simulink library "sm_wheel_loader_lib"  (R2026a)
settings: Solver=VariableStepAuto
undefined symbols (not defined in the file): AToTOrificeVector, BiPOrificeVector, boomHEArea, boomREArea, BToTOrificeVector, fluids, GRake, GToothL, GToothR, HMPST, HydFcnParams, logLoad, Position, PToAOrificeVector, PToBOrificeVector, RakeL, RakeR, testInput, Wheel_Loader, X, Y, Z
libraries: sm_lib x694, fl_lib x183, nesl_utility x74, SimscapeFluids_lib x62, sdl_lib x25, cvt_components_lib x25, simulink_extras x5, $bdroot x4, wheel_loader_contact_lib x4, ee_lib x2, SignalEditorBlockLib x1, batteryecm_lib x1
(part 9 of 25)

== system sm_wheel_loader_lib/Wheel Loader Vehicle/Steering Actuator/Cylinder ==
  Collar : sm_lib/Body Elements/File Solid  ExtGeomFileName=Steer_Act_Cylinder_Collar.STEP  UnitType=FromFile  ExtGeomFileUnits=m  StepReaderType=HEX  ExportConvexHullGeometry=off  InertiaType=Custom  BasedOnType=DensityFromFile  Density=1000  DensityUnits=kg/m^3  Mass=Wheel_Loader.bodyGroups(50).subGroups(3).inertialProperties.mass  MassUnits=kg  CenterOfMass=Wheel_Loader.bodyGroups(50).subGroups(3).inertialProperties.centerOfMass  CenterOfMassUnits=m  MomentsOfInertia=Wheel_Loader.bodyGroups(50).subGroups(3).inertialProperties.momentsOfInertia  MomentsOfInertiaUnits=kg*m^2  ProductsOfInertia=Wheel_Loader.bodyGroups(50).subGroups(3).inertialProperties.productsOfInertia  ProductsOfInertiaUnits=kg*m^2  GraphicType=FromGeometry  MarkerShape=Sphere  MarkerSize=10  GraphicVisPropType=SimpleVisualProperties  GraphicDiffuseColor=Wheel_Loader.bodyGroups(50).subGroups(3).visualProperties.rgb  GraphicOpacity=Wheel_Loader.bodyGroups(50).subGroups(3).visualProperties.opacity  GraphicSpecularColor=[0.5 0.5 0.5 1.0]  GraphicAmbientColor=[0.15 0.15 0.15 1.0]  GraphicEmissiveColor=[0.0 0.0 0.0 1.0]  GraphicShininess=75  DoExposeReferenceFrame=on  SerializedFrames=<Frames/>
  Cylinder : sm_lib/Body Elements/File Solid  ExtGeomFileName=Steer_Act_Cylinder.STEP  UnitType=FromFile  ExtGeomFileUnits=m  StepReaderType=HEX  ExportConvexHullGeometry=off  InertiaType=Custom  BasedOnType=DensityFromFile  Density=1000  DensityUnits=kg/m^3  Mass=Wheel_Loader.bodyGroups(50).subGroups(1).inertialProperties.mass  MassUnits=kg  CenterOfMass=Wheel_Loader.bodyGroups(50).subGroups(1).inertialProperties.centerOfMass  CenterOfMassUnits=m  MomentsOfInertia=Wheel_Loader.bodyGroups(50).subGroups(1).inertialProperties.momentsOfInertia  MomentsOfInertiaUnits=kg*m^2  ProductsOfInertia=Wheel_Loader.bodyGroups(50).subGroups(1).inertialProperties.productsOfInertia  ProductsOfInertiaUnits=kg*m^2  GraphicType=FromGeometry  MarkerShape=Sphere  MarkerSize=10  GraphicVisPropType=SimpleVisualProperties  GraphicDiffuseColor=Wheel_Loader.bodyGroups(50).subGroups(1).visualProperties.rgb  GraphicOpacity=Wheel_Loader.bodyGroups(50).subGroups(1).visualProperties.opacity  GraphicSpecularColor=[0.5 0.5 0.5 1.0]  GraphicAmbientColor=[0.15 0.15 0.15 1.0]  GraphicEmissiveColor=[0.0 0.0 0.0 1.0]  GraphicShininess=75  DoExposeReferenceFrame=on  SerializedFrames=<Frames/>
  RT_RearFrame_SteeringActCyl : sm_lib/Frames and Transforms/Rigid Transform  RotationMethod=RotationMatrix  FollAlignAxisA=+X  BaseAlignAxisA=+Y  FollAlignAxisB=+Y  BaseAlignAxisB=+Z  RotationStandardAxis=+Z  RotationAngle=0.0  RotationAngleUnits=deg  RotationArbitraryAxis=[0 0 1]  RotationSequenceAxes=FollowerAxes  RotationSequence=XYX  RotationSequenceAngles=[0 0 0]  RotationSequenceAnglesUnits=deg  RotationMatrix=Wheel_Loader.coordSys(23).transform.rotation  Quaternion=[1 0 0 0]  TranslationMethod=Cartesian  TranslationCartesianOffset=Wheel_Loader.coordSys(23).transform.translation  TranslationCartesianOffsetUnits=m  TranslationStandardAxis=+Z  TranslationStandardOffset=0  TranslationStandardOffsetUnits=m  TranslationROffset=0  TranslationROffsetUnits=m  TranslationThetaOffset=0  TranslationThetaOffsetUnits=deg  TranslationZOffset=0  TranslationZOffsetUnits=m
  RT_Steering_Actuator : sm_lib/Frames and Transforms/Rigid Transform  RotationMethod=RotationMatrix  FollAlignAxisA=+X  BaseAlignAxisA=+Y  FollAlignAxisB=+Y  BaseAlignAxisB=+Z  RotationStandardAxis=+Z  RotationAngle=0.0  RotationAngleUnits=deg  RotationArbitraryAxis=[0 0 1]  RotationSequenceAxes=FollowerAxes  RotationSequence=XYX  RotationSequenceAngles=[0 0 0]  RotationSequenceAnglesUnits=deg  RotationMatrix=Wheel_Loader.coordSys(24).transform.rotation  Quaternion=[1 0 0 0]  TranslationMethod=Cartesian  TranslationCartesianOffset=Wheel_Loader.coordSys(24).transform.translation  TranslationCartesianOffsetUnits=m  TranslationStandardAxis=+Z  TranslationStandardOffset=0  TranslationStandardOffsetUnits=m  TranslationROffset=0  TranslationROffsetUnits=m  TranslationThetaOffset=0  TranslationThetaOffsetUnits=deg  TranslationZOffset=0  TranslationZOffsetUnits=m
  RT_Steering_Actuator_Offset : sm_lib/Frames and Transforms/Rigid Transform  RotationMethod=None  FollAlignAxisA=+X  BaseAlignAxisA=+Y  FollAlignAxisB=+Y  BaseAlignAxisB=+Z  RotationStandardAxis=+Z  RotationAngle=0.0  RotationAngleUnits=deg  RotationArbitraryAxis=[0 0 1]  RotationSequenceAxes=FollowerAxes  RotationSequence=XYX  RotationSequenceAngles=[0 0 0]  RotationSequenceAnglesUnits=deg  RotationMatrix=[1 0 0; 0 1 0; 0 0 1]  Quaternion=[1 0 0 0]  TranslationMethod=StandardAxis  TranslationCartesianOffset=[0 0 0]  TranslationCartesianOffsetUnits=m  TranslationStandardAxis=+Z  TranslationStandardOffset=HydFcnParams.steerActuator.mechModelCylOffset  TranslationStandardOffsetUnits=mm  TranslationROffset=0  TranslationROffsetUnits=m  TranslationThetaOffset=0  TranslationThetaOffsetUnits=deg  TranslationZOffset=0  TranslationZOffsetUnits=m
  Seal : sm_lib/Body Elements/File Solid  ExtGeomFileName=Steer_Act_Cylinder_Seal.STEP  UnitType=FromFile  ExtGeomFileUnits=m  StepReaderType=HEX  ExportConvexHullGeometry=off  InertiaType=Custom  BasedOnType=DensityFromFile  Density=1000  DensityUnits=kg/m^3  Mass=Wheel_Loader.bodyGroups(50).subGroups(2).inertialProperties.mass  MassUnits=kg  CenterOfMass=Wheel_Loader.bodyGroups(50).subGroups(2).inertialProperties.centerOfMass  CenterOfMassUnits=m  MomentsOfInertia=Wheel_Loader.bodyGroups(50).subGroups(2).inertialProperties.momentsOfInertia  MomentsOfInertiaUnits=kg*m^2  ProductsOfInertia=Wheel_Loader.bodyGroups(50).subGroups(2).inertialProperties.productsOfInertia  ProductsOfInertiaUnits=kg*m^2  GraphicType=FromGeometry  MarkerShape=Sphere  MarkerSize=10  GraphicVisPropType=SimpleVisualProperties  GraphicDiffuseColor=Wheel_Loader.bodyGroups(50).subGroups(2).visualProperties.rgb  GraphicOpacity=Wheel_Loader.bodyGroups(50).subGroups(2).visualProperties.opacity  GraphicSpecularColor=[0.5 0.5 0.5 1.0]  GraphicAmbientColor=[0.15 0.15 0.15 1.0]  GraphicEmissiveColor=[0.0 0.0 0.0 1.0]  GraphicShininess=75  DoExposeReferenceFrame=on  SerializedFrames=<Frames/>
  B : PMIOPort  Side=Left
  F : PMIOPort  Port=2  Side=Right
  connections:
  Seal/RConn1 -- Collar/RConn1 -- Cylinder/RConn1 -- RT_RearFrame_SteeringActCyl/LConn1 -- RT_Steering_Actuator/LConn1
  RT_RearFrame_SteeringActCyl/RConn1 -- B/RConn1
  RT_Steering_Actuator_Offset/RConn1 -- F/RConn1
  RT_Steering_Actuator/RConn1 -- RT_Steering_Actuator_Offset/LConn1

== system sm_wheel_loader_lib/Wheel Loader Vehicle/Steering Actuator/Rod ==
  Collar : sm_lib/Body Elements/File Solid  ExtGeomFileName=Steer_Act_Rod_Collar.STEP  UnitType=FromFile  ExtGeomFileUnits=m  StepReaderType=HEX  ExportConvexHullGeometry=off  InertiaType=Custom  BasedOnType=DensityFromFile  Density=1000  DensityUnits=kg/m^3  Mass=Wheel_Loader.bodyGroups(51).subGroups(2).inertialProperties.mass  MassUnits=kg  CenterOfMass=Wheel_Loader.bodyGroups(51).subGroups(2).inertialProperties.centerOfMass  CenterOfMassUnits=m  MomentsOfInertia=Wheel_Loader.bodyGroups(51).subGroups(2).inertialProperties.momentsOfInertia  MomentsOfInertiaUnits=kg*m^2  ProductsOfInertia=Wheel_Loader.bodyGroups(51).subGroups(2).inertialProperties.productsOfInertia  ProductsOfInertiaUnits=kg*m^2  GraphicType=FromGeometry  MarkerShape=Sphere  MarkerSize=10  GraphicVisPropType=SimpleVisualProperties  GraphicDiffuseColor=Wheel_Loader.bodyGroups(51).subGroups(2).visualProperties.rgb  GraphicOpacity=Wheel_Loader.bodyGroups(51).subGroups(2).visualProperties.opacity  GraphicSpecularColor=[0.5 0.5 0.5 1.0]  GraphicAmbientColor=[0.15 0.15 0.15 1.0]  GraphicEmissiveColor=[0.0 0.0 0.0 1.0]  GraphicShininess=75  DoExposeReferenceFrame=on  SerializedFrames=<Frames/>
  RT_SteeringActRod_FrontFrame : sm_lib/Frames and Transforms/Rigid Transform  RotationMethod=RotationMatrix  FollAlignAxisA=+X  BaseAlignAxisA=+Y  FollAlignAxisB=+Y  BaseAlignAxisB=+Z  RotationStandardAxis=+Z  RotationAngle=0.0  RotationAngleUnits=deg  RotationArbitraryAxis=[0 0 1]  RotationSequenceAxes=FollowerAxes  RotationSequence=XYX  RotationSequenceAngles=[0 0 0]  RotationSequenceAnglesUnits=deg  RotationMatrix=Wheel_Loader.coordSys(25).transform.rotation  Quaternion=[1 0 0 0]  TranslationMethod=Cartesian  TranslationCartesianOffset=Wheel_Loader.coordSys(25).transform.translation  TranslationCartesianOffsetUnits=m  TranslationStandardAxis=+Z  TranslationStandardOffset=0  TranslationStandardOffsetUnits=m  TranslationROffset=0  TranslationROffsetUnits=m  TranslationThetaOffset=0  TranslationThetaOffsetUnits=deg  TranslationZOffset=0  TranslationZOffsetUnits=m
  RT_Steering_Actuator : sm_lib/Frames and Transforms/Rigid Transform  RotationMethod=RotationMatrix  FollAlignAxisA=+X  BaseAlignAxisA=+Y  FollAlignAxisB=+Y  BaseAlignAxisB=+Z  RotationStandardAxis=+Z  RotationAngle=0.0  RotationAngleUnits=deg  RotationArbitraryAxis=[0 0 1]  RotationSequenceAxes=FollowerAxes  RotationSequence=XYX  RotationSequenceAngles=[0 0 0]  RotationSequenceAnglesUnits=deg  RotationMatrix=Wheel_Loader.coordSys(24).transform.rotation  Quaternion=[1 0 0 0]  TranslationMethod=Cartesian  TranslationCartesianOffset=Wheel_Loader.coordSys(24).transform.translation  TranslationCartesianOffsetUnits=m  TranslationStandardAxis=+Z  TranslationStandardOffset=0  TranslationStandardOffsetUnits=m  TranslationROffset=0  TranslationROffsetUnits=m  TranslationThetaOffset=0  TranslationThetaOffsetUnits=deg  TranslationZOffset=0  TranslationZOffsetUnits=m
  RT_Steering_Actuator_Offset : sm_lib/Frames and Transforms/Rigid Transform  RotationMethod=None  FollAlignAxisA=+X  BaseAlignAxisA=+Y  FollAlignAxisB=+Y  BaseAlignAxisB=+Z  RotationStandardAxis=+Z  RotationAngle=0.0  RotationAngleUnits=deg  RotationArbitraryAxis=[0 0 1]  RotationSequenceAxes=FollowerAxes  RotationSequence=XYX  RotationSequenceAngles=[0 0 0]  RotationSequenceAnglesUnits=deg  RotationMatrix=[1 0 0; 0 1 0; 0 0 1]  Quaternion=[1 0 0 0]  TranslationMethod=StandardAxis  TranslationCartesianOffset=[0 0 0]  TranslationCartesianOffsetUnits=m  TranslationStandardAxis=+Z  TranslationStandardOffset=HydFcnParams.steerActuator.mechModelRodOffset  TranslationStandardOffsetUnits=mm  TranslationROffset=0  TranslationROffsetUnits=m  TranslationThetaOffset=0  TranslationThetaOffsetUnits=deg  TranslationZOffset=0  TranslationZOffsetUnits=m
  Rod : sm_lib/Body Elements/File Solid  ExtGeomFileName=Steer_Act_Rod.STEP  UnitType=FromFile  ExtGeomFileUnits=m  StepReaderType=HEX  ExportConvexHullGeometry=off  InertiaType=Custom  BasedOnType=DensityFromFile  Density=1000  DensityUnits=kg/m^3  Mass=Wheel_Loader.bodyGroups(51).subGroups(1).inertialProperties.mass  MassUnits=kg  CenterOfMass=Wheel_Loader.bodyGroups(51).subGroups(1).inertialProperties.centerOfMass  CenterOfMassUnits=m  MomentsOfInertia=Wheel_Loader.bodyGroups(51).subGroups(1).inertialProperties.momentsOfInertia  MomentsOfInertiaUnits=kg*m^2  ProductsOfInertia=Wheel_Loader.bodyGroups(51).subGroups(1).inertialProperties.productsOfInertia  ProductsOfInertiaUnits=kg*m^2  GraphicType=FromGeometry  MarkerShape=Sphere  MarkerSize=10  GraphicVisPropType=SimpleVisualProperties  GraphicDiffuseColor=Wheel_Loader.bodyGroups(51).subGroups(1).visualProperties.rgb  GraphicOpacity=Wheel_Loader.bodyGroups(51).subGroups(1).visualProperties.opacity  GraphicSpecularColor=[0.5 0.5 0.5 1.0]  GraphicAmbientColor=[0.15 0.15 0.15 1.0]  GraphicEmissiveColor=[0.0 0.0 0.0 1.0]  GraphicShininess=75  DoExposeReferenceFrame=on  SerializedFrames=<Frames/>
  B : PMIOPort  Side=Left
  F : PMIOPort  Port=2  Side=Right
  connections:
  RT_Steering_Actuator/LConn1 -- Collar/RConn1 -- Rod/RConn1 -- RT_SteeringActRod_FrontFrame/LConn1
  RT_Steering_Actuator_Offset/RConn1 -- B/RConn1
  RT_SteeringActRod_FrontFrame/RConn1 -- F/RConn1
  RT_Steering_Actuator/RConn1 -- RT_Steering_Actuator_Offset/LConn1

== system sm_wheel_loader_lib/Controller/Desired Ratio Calc/HRB Control/PI HRB Brake ==
  error : Inport
  Rset : Inport  Port=2
  Gain : Gain  Gain=0.02*0.2
  Gain3 : Gain  Gain=0.002+0.0005
  Integrator : Integrator  ExternalReset=falling
  Sum : Sum  Inputs=++|
  ctrl : Outport
  wires:
  Rset/1 -> Integrator/2
  Integrator/1 -> Sum/1
  error/1 -> Gain3/1, Gain/1
  Sum/1 -> ctrl/1
  Gain3/1 -> Integrator/1
  Gain/1 -> Sum/2

== system sm_wheel_loader_lib/Controller/Desired Ratio Calc/HRB Control/PI HRB Regen ==
  error : Inport
  Rset : Inport  Port=2
  Gain : Gain  Gain=0.01*0.2
  Gain3 : Gain  Gain=0.001
  Integrator : Integrator  ExternalReset=falling
  Sum : Sum  Inputs=++|
  ctrl : Outport
  wires:
  Gain/1 -> Sum/2
  Gain3/1 -> Integrator/1
  Sum/1 -> ctrl/1
  error/1 -> Gain/1, Gain3/1
  Integrator/1 -> Sum/1
  Rset/1 -> Integrator/2

== system sm_wheel_loader_lib/Controller/Desired Ratio Calc/MB Control/PI MB No HRB ==
  error : Inport
  Rset : Inport  Port=2
  Gain : Gain  Gain=0.01
  Gain3 : Gain  Gain=0.002
  Integrator : Integrator  ExternalReset=falling
  Sum : Sum  Inputs=++|
  ctrl : Outport
  wires:
  Rset/1 -> Integrator/2
  Integrator/1 -> Sum/1
  error/1 -> Gain3/1, Gain/1
  Sum/1 -> ctrl/1
  Gain3/1 -> Integrator/1
  Gain/1 -> Sum/2

== system sm_wheel_loader_lib/Controller/Desired Ratio Calc/MB Control/PI MB with MRB ==
  error : Inport
  Rset : Inport  Port=2
  Gain : Gain  Gain=0.005
  Gain3 : Gain  Gain=0.002
  Integrator : Integrator  ExternalReset=falling
  Sum : Sum  Inputs=++|
  ctrl : Outport
  wires:
  Gain/1 -> Sum/2
  Gain3/1 -> Integrator/1
  Sum/1 -> ctrl/1
  error/1 -> Gain/1, Gain3/1
  Integrator/1 -> Sum/1
  Rset/1 -> Integrator/2

== system sm_wheel_loader_lib/Wheel Loader Vehicle/Actuators/Hydraulic/Actuator Linkage ==
  Actuator LiftL : SimscapeFluids_lib/Isothermal Liquid/Actuators/Double-Acting Actuator (IL)  single_fluid=true  mech_orientation=foundation.enum.MechOrientationTranslational.Positive  piston_area_A=HydFcnParams.liftActuator.headEndArea mm^2  piston_area_B=HydFcnParams.liftActuator.rodEndArea mm^2  stroke=HydFcnParams.liftActuator.stroke mm  dead_volume_A=1e-4 m^3  dead_volume_B=1e-4 m^3  pressure_spec=foundation.enum.pressure_spec.atmospheric  environment_pressure=0.101325 MPa  hardstop_model=simscape.enum.hardstop.smooth  stiff_coeff=1e8 N/m  damping_coeff=1e5 N/(m/s)  transition=0.1 mm  coeff_rest=0.7  v_tol=0.001 m/s  f_tol=0.001 N  cushion_A_spec=simscape.enum.onoff.off  area_plunger_A=boomHEArea/4 mm^2  length_plunger_A=5 mm  area_cushion_orifice_A=5 mm^2  area_leak_plunger_A=1e-7 m^2  p_crack_differential_A=0.01 MPa  press_max_differential_A=0.1 MPa  check_valve_area_max_A=1e-4 m^2  check_valve_area_leak_A=1e-10 m^2  smoothing_factor_A=0  cushion_B_spec=simscape.enum.onoff.off  area_plunger_B=boomREArea/4 mm^2  length_plunger_B=5 mm  area_cushion_orifice_B=5 mm^2  area_leak_plunger_B=1e-7 m^2  p_crack_differential_B=0.01 MPa  press_max_differential_B=0.1 MPa  check_valve_area_max_B=1e-4 m^2  check_valve_area_leak_B=1e-10 m^2  smoothing_factor_B=0  friction_spec=simscape.enum.onoff.on  breakaway_Coulomb_ratio=HydFcnParams.liftActuator.brkawyToCoulRatio  breakaway_velocity=HydFcnParams.liftActuator.brkawyVel m/s  preload_force=HydFcnParams.liftActuator.preloadForce N  Coulomb_coeff=HydFcnParams.liftActuator.coulForceCoef N/Pa  viscous_coeff=HydFcnParams.liftActuator.viscCoeff N/(m/s)  leakage_spec=simscape.enum.onoff.off  clearance=1e-4 m  piston_length=0.01 m  displacement_spec=foundation.enum.DisplacementSpec.Calculate  x0=testInput.Active.Lift.p(1)*1000 mm  dynamic_compressibility=simscape.enum.onoff.on  p0_A=HydFcnParams.liftActuator.initHEPr bar  p0_B=HydFcnParams.liftActuator.initREPr bar  p_nominal_A=0.101325 MPa  p_nominal_B=0.101325 MPa
  Actuator LiftR : SimscapeFluids_lib/Isothermal Liquid/Actuators/Double-Acting Actuator (IL)  single_fluid=true  mech_orientation=foundation.enum.MechOrientationTranslational.Positive  piston_area_A=HydFcnParams.liftActuator.headEndArea mm^2  piston_area_B=HydFcnParams.liftActuator.rodEndArea mm^2  stroke=HydFcnParams.liftActuator.stroke mm  dead_volume_A=1e-4 m^3  dead_volume_B=1e-4 m^3  pressure_spec=foundation.enum.pressure_spec.atmospheric  environment_pressure=0.101325 MPa  hardstop_model=simscape.enum.hardstop.smooth  stiff_coeff=1e8 N/m  damping_coeff=1e5 N/(m/s)  transition=0.1 mm  coeff_rest=0.7  v_tol=0.001 m/s  f_tol=0.001 N  cushion_A_spec=simscape.enum.onoff.off  area_plunger_A=boomHEArea/4 mm^2  length_plunger_A=5 mm  area_cushion_orifice_A=5 mm^2  area_leak_plunger_A=1e-7 m^2  p_crack_differential_A=0.01 MPa  press_max_differential_A=0.1 MPa  check_valve_area_max_A=1e-4 m^2  check_valve_area_leak_A=1e-10 m^2  smoothing_factor_A=0  cushion_B_spec=simscape.enum.onoff.off  area_plunger_B=boomREArea/4 mm^2  length_plunger_B=5 mm  area_cushion_orifice_B=5 mm^2  area_leak_plunger_B=1e-7 m^2  p_crack_differential_B=0.01 MPa  press_max_differential_B=0.1 MPa  check_valve_area_max_B=1e-4 m^2  check_valve_area_leak_B=1e-10 m^2  smoothing_factor_B=0  friction_spec=simscape.enum.onoff.on  breakaway_Coulomb_ratio=HydFcnParams.liftActuator.brkawyToCoulRatio  breakaway_velocity=HydFcnParams.liftActuator.brkawyVel m/s  preload_force=HydFcnParams.liftActuator.preloadForce N  Coulomb_coeff=HydFcnParams.liftActuator.coulForceCoef N/Pa  viscous_coeff=HydFcnParams.liftActuator.viscCoeff N/(m/s)  leakage_spec=simscape.enum.onoff.off  clearance=1e-4 m  piston_length=0.01 m  displacement_spec=foundation.enum.DisplacementSpec.Calculate  x0=testInput.Active.Lift.p(1)*1000 mm  dynamic_compressibility=simscape.enum.onoff.on  p0_A=HydFcnParams.liftActuator.initHEPr bar  p0_B=HydFcnParams.liftActuator.initREPr bar  p_nominal_A=0.101325 MPa  p_nominal_B=0.101325 MPa
  Actuator Tilt : SimscapeFluids_lib/Isothermal Liquid/Actuators/Double-Acting Actuator (IL)  single_fluid=true  mech_orientation=foundation.enum.MechOrientationTranslational.Positive  piston_area_A=HydFcnParams.tiltActuator.headEndArea mm^2  piston_area_B=HydFcnParams.tiltActuator.rodEndArea mm^2  stroke=HydFcnParams.tiltActuator.stroke mm  dead_volume_A=1e-4 m^3  dead_volume_B=1e-4 m^3  pressure_spec=foundation.enum.pressure_spec.atmospheric  environment_pressure=0.101325 MPa  hardstop_model=simscape.enum.hardstop.smooth  stiff_coeff=1e8 N/m  damping_coeff=1e5 N/(m/s)  transition=0.1 mm  coeff_rest=0.7  v_tol=0.001 m/s  f_tol=0.001 N  cushion_A_spec=simscape.enum.onoff.off  area_plunger_A=boomHEArea/4 mm^2  length_plunger_A=5 mm  area_cushion_orifice_A=5 mm^2  area_leak_plunger_A=1e-7 m^2  p_crack_differential_A=0.01 MPa  press_max_differential_A=0.1 MPa  check_valve_area_max_A=1e-4 m^2  check_valve_area_leak_A=1e-10 m^2  smoothing_factor_A=0  cushion_B_spec=simscape.enum.onoff.off  area_plunger_B=boomREArea/4 mm^2  length_plunger_B=5 mm  area_cushion_orifice_B=5 mm^2  area_leak_plunger_B=1e-7 m^2  p_crack_differential_B=0.01 MPa  press_max_differential_B=0.1 MPa  check_valve_area_max_B=1e-4 m^2  check_valve_area_leak_B=1e-10 m^2  smoothing_factor_B=0  friction_spec=true  breakaway_Coulomb_ratio=HydFcnParams.tiltActuator.brkawyToCoulRatio  breakaway_velocity=HydFcnParams.tiltActuator.brkawyVel m/s  preload_force=HydFcnParams.tiltActuator.preloadForce N  Coulomb_coeff=HydFcnParams.tiltActuator.coulForceCoef N/Pa  viscous_coeff=HydFcnParams.tiltActuator.viscCoeff lbf/(in/s)  leakage_spec=simscape.enum.onoff.off  clearance=1e-4 m  piston_length=0.01 m  displacement_spec=foundation.enum.DisplacementSpec.Calculate  x0=testInput.Active.Tilt.p(1)*1000 mm  dynamic_compressibility=simscape.enum.onoff.on  p0_A=HydFcnParams.tiltActuator.initHEPr bar  p0_B=HydFcnParams.tiltActuator.initREPr bar  p_nominal_A=0.101325 MPa  p_nominal_B=0.101325 MPa
  MTRef Tilt : fl_lib/Mechanical/Translational Elements/Mechanical Translational Reference
  MTRef Tilt LiftR : fl_lib/Mechanical/Translational Elements/Mechanical Translational Reference
  MTRef TiltL : fl_lib/Mechanical/Translational Elements/Mechanical Translational Reference
  PS Terminator : fl_lib/Physical Signals/Sinks/PS Terminator
  PS Terminator1 : fl_lib/Physical Signals/Sinks/PS Terminator
  PS Terminator2 : fl_lib/Physical Signals/Sinks/PS Terminator
  LA : PMIOPort  Side=Left
  LB : PMIOPort  Port=2  Side=Left
  TA : PMIOPort  Port=3  Side=Left
  TB : PMIOPort  Port=4  Side=Left
  RLiftL : PMIOPort  Port=5  Side=Right
  RLiftR : PMIOPort  Port=6  Side=Right
  RTilt : PMIOPort  Port=7  Side=Right
  connections:
  Actuator Tilt/LConn2 -- TA/RConn1
  Actuator Tilt/RConn3 -- TB/RConn1
  RLiftR/RConn1 -- Actuator LiftR/RConn2
  Actuator LiftR/RConn3 -- Actuator LiftL/RConn3 -- LB/RConn1
  Actuator LiftR/LConn2 -- Actuator LiftL/LConn2 -- LA/RConn1
  Actuator LiftL/LConn1 -- MTRef TiltL/LConn1
  RLiftL/RConn1 -- Actuator LiftL/RConn2
  MTRef Tilt/LConn1 -- Actuator Tilt/LConn1
  RTilt/RConn1 -- Actuator Tilt/RConn2
  MTRef Tilt LiftR/LConn1 -- Actuator LiftR/LConn1
  Actuator LiftL/RConn1 -- PS Terminator/LConn1
  PS Terminator1/LConn1 -- Actuator LiftR/RConn1
  Actuator Tilt/RConn1 -- PS Terminator2/LConn1

== system sm_wheel_loader_lib/Wheel Loader Vehicle/Actuators/Hydraulic/Actuator Steer ==
  Actuator Steer : SimscapeFluids_lib/Isothermal Liquid/Actuators/Double-Acting Actuator (IL)  single_fluid=true  mech_orientation=foundation.enum.MechOrientationTranslational.Positive  piston_area_A=HydFcnParams.steerActuator.headEndArea mm^2  piston_area_B=HydFcnParams.steerActuator.rodEndArea mm^2  stroke=HydFcnParams.steerActuator.stroke mm  dead_volume_A=1e-4 m^3  dead_volume_B=1e-4 m^3  pressure_spec=foundation.enum.pressure_spec.atmospheric  environment_pressure=0.101325 MPa  hardstop_model=simscape.enum.hardstop.smooth  stiff_coeff=1e8 N/m  damping_coeff=1e5 N/(m/s)  transition=0.1 mm  coeff_rest=0.7  v_tol=0.001 m/s  f_tol=0.001 N  cushion_A_spec=simscape.enum.onoff.off  area_plunger_A=boomHEArea/4 mm^2  length_plunger_A=5 mm  area_cushion_orifice_A=5 mm^2  area_leak_plunger_A=1e-7 m^2  p_crack_differential_A=0.01 MPa  press_max_differential_A=0.1 MPa  check_valve_area_max_A=1e-4 m^2  check_valve_area_leak_A=1e-10 m^2  smoothing_factor_A=0  cushion_B_spec=simscape.enum.onoff.off  area_plunger_B=boomREArea/4 mm^2  length_plunger_B=5 mm  area_cushion_orifice_B=5 mm^2  area_leak_plunger_B=1e-7 m^2  p_crack_differential_B=0.01 MPa  press_max_differential_B=0.1 MPa  check_valve_area_max_B=1e-4 m^2  check_valve_area_leak_B=1e-10 m^2  smoothing_factor_B=0  friction_spec=simscape.enum.onoff.on  breakaway_Coulomb_ratio=HydFcnParams.steerActuator.brkawyToCoulRatio  breakaway_velocity=HydFcnParams.steerActuator.brkawyVel m/s  preload_force=HydFcnParams.steerActuator.preloadForce N  Coulomb_coeff=HydFcnParams.steerActuator.coulForceCoef N/Pa  viscous_coeff=HydFcnParams.steerActuator.viscCoeff lbf/(in/s)  leakage_spec=simscape.enum.onoff.off  clearance=1e-4 m  piston_length=0.01 m  displacement_spec=foundation.enum.DisplacementSpec.Calculate  x0=testInput.Active.Steer.p(1)*1000 mm  dynamic_compressibility=simscape.enum.onoff.on  p0_A=HydFcnParams.steerActuator.initHEPr bar  p0_B=HydFcnParams.steerActuator.initREPr bar  p_nominal_A=0.101325 MPa  p_nominal_B=0.101325 MPa
  MTRef : fl_lib/Mechanical/Translational Elements/Mechanical Translational Reference
  PS Terminator : fl_lib/Physical Signals/Sinks/PS Terminator
  A : PMIOPort  Side=Left
  B : PMIOPort  Port=2  Side=Left
  R : PMIOPort  Port=3  Side=Right
  connections:
  Actuator Steer/LConn1 -- MTRef/LConn1
  A/RConn1 -- Actuator Steer/LConn2
  B/RConn1 -- Actuator Steer/RConn3
  R/RConn1 -- Actuator Steer/RConn2
  Actuator Steer/RConn1 -- PS Terminator/LConn1

== system sm_wheel_loader_lib/Wheel Loader Vehicle/Actuators/Hydraulic/Controller ==
  note: Inputs - Outputs:
      |
      | Joystick position for lift (-1 to 1) velocity control - lift arm spool position
      | Joystick position for tilt (-1 to 1) velocity control - tilt spool position
  BusElementIn : Inport  PortName=Cmd  Element=LiftCmd
  BusElementIn1 : Inport  PortName=Cmd  Element=TiltCmd
  Gain : Gain  Gain=5
  Gain1 : Gain  Gain=5
  LiftSpoolPosCmdRateLimit : RateLimiter  RisingSlewLimit=HydFcnParams.liftActCtrl.posSpoolCmdRateLimit  FallingSlewLimit=HydFcnParams.liftActCtrl.negSpoolCmdRateLimit  SampleTimeMode=inherited
  LiftSpoolPosCmdSaturation : Saturate  UpperLimit=HydFcnParams.liftActCtrl.maxSpoolCmd  LowerLimit=HydFcnParams.liftActCtrl.minSpoolCmd
  TiltSpoolPosCmdRateLimit : RateLimiter  RisingSlewLimit=HydFcnParams.tiltActCtrl.posSpoolCmdRateLimit  FallingSlewLimit=HydFcnParams.tiltActCtrl.negSpoolCmdRateLimit  SampleTimeMode=inherited
  TiltSpoolPosCmdSaturation : Saturate  UpperLimit=HydFcnParams.tiltActCtrl.maxSpoolCmd  LowerLimit=HydFcnParams.tiltActCtrl.minSpoolCmd
  Out Bus Element : Outport  PortName=pSpool  Element=tilt
  Out Bus Element1 : Outport  PortName=pSpool  Element=lift
  wires:
  Gain/1 -> LiftSpoolPosCmdSaturation/1
  Gain1/1 -> TiltSpoolPosCmdSaturation/1
  LiftSpoolPosCmdSaturation/1 -> LiftSpoolPosCmdRateLimit/1
  TiltSpoolPosCmdSaturation/1 -> TiltSpoolPosCmdRateLimit/1
  LiftSpoolPosCmdRateLimit/1 -> Out Bus Element1/1  "LiftSpoolPosCmd"
  TiltSpoolPosCmdRateLimit/1 -> Out Bus Element/1  "TiltSpoolCmd"
  BusElementIn1/1 -> Gain1/1
  BusElementIn/1 -> Gain/1

== system sm_wheel_loader_lib/Wheel Loader Vehicle/Actuators/Hydraulic/Implement ==
  A : Inport
  Bucket : Subsystem  VariantControl=Bucket
      mask Display: image('sm_wheel_loader_actuator_bucket_IMAGE.png')
  Grapple : Subsystem  VariantControl=Grapple
      mask Display: image('sm_wheel_loader_actuator_grapple_IMAGE.png')
  Impl : PMIOPort  Side=Right

== system sm_wheel_loader_lib/Wheel Loader Vehicle/Actuators/Hydraulic/Valve Steer ==
  CV SteerA : SimscapeFluids_lib/Isothermal Liquid/Valves & Orifices/Directional Control Valves/Check Valve (IL)  opening_spec=2*(fluids.isothermal_liquid.valves_orifices.enum.opening_spec.linear)-1  pressure_control_spec=fluids.isothermal_liquid.valves_orifices.enum.pressure_control_spec.dp  p_crack_differential=HydFcnParams.checkValves.crackingPrDiff bar  p_crack_gauge=0.1 MPa  press_max_differential=HydFcnParams.checkValves.maxOpeningPrDiff bar  press_max_gauge=0.2 MPa  area_max=HydFcnParams.checkValves.maxOpeningArea mm^2  area_leak="HydFcnParams.checkValves.leakageArea  mm^2"  p_diff_TLU=[0.01 : 0.01 : 0.1] MPa  valve_area_TLU=[1e-10, 1e-05, 2e-05, 3e-05, 4e-05, 5e-05, 6e-05, 7.5e-05, 8.5e-05, .0001] m^2  vol_flow_TLU=[.000358, .045, .11, .191, .284, .39, .505, .63, .764, .905] .* 1e-3 m^3/s  area=inf m^2  Cd=HydFcnParams.checkValves.dischargeCoef  Re_c=HydFcnParams.checkValves.critReynoldsNmbr  smoothing_factor=HydFcnParams.checkValves.smoothingFactor  pressure_recovery=simscape.enum.onoff.off  opening_dynamics=simscape.enum.onoff.off  tau=0.1 s
  CV SteerB : SimscapeFluids_lib/Isothermal Liquid/Valves & Orifices/Directional Control Valves/Check Valve (IL)  opening_spec=2*(fluids.isothermal_liquid.valves_orifices.enum.opening_spec.linear)-1  pressure_control_spec=fluids.isothermal_liquid.valves_orifices.enum.pressure_control_spec.dp  p_crack_differential=HydFcnParams.checkValves.crackingPrDiff bar  p_crack_gauge=0.1 MPa  press_max_differential=HydFcnParams.checkValves.maxOpeningPrDiff bar  press_max_gauge=0.2 MPa  area_max=HydFcnParams.checkValves.maxOpeningArea mm^2  area_leak="HydFcnParams.checkValves.leakageArea  mm^2"  p_diff_TLU=[0.01 : 0.01 : 0.1] MPa  valve_area_TLU=[1e-10, 1e-05, 2e-05, 3e-05, 4e-05, 5e-05, 6e-05, 7.5e-05, 8.5e-05, .0001] m^2  vol_flow_TLU=[.000358, .045, .11, .191, .284, .39, .505, .63, .764, .905] .* 1e-3 m^3/s  area=inf m^2  Cd=HydFcnParams.checkValves.dischargeCoef  Re_c=HydFcnParams.checkValves.critReynoldsNmbr  smoothing_factor=HydFcnParams.checkValves.smoothingFactor  pressure_recovery=simscape.enum.onoff.off  opening_dynamics=simscape.enum.onoff.off  tau=0.1 s
  CV SteerP : SimscapeFluids_lib/Isothermal Liquid/Valves & Orifices/Directional Control Valves/Check Valve (IL)  opening_spec=2*(fluids.isothermal_liquid.valves_orifices.enum.opening_spec.linear)-1  pressure_control_spec=fluids.isothermal_liquid.valves_orifices.enum.pressure_control_spec.dp  p_crack_differential=HydFcnParams.checkValves.crackingPrDiff bar  p_crack_gauge=0.1 MPa  press_max_differential=HydFcnParams.checkValves.maxOpeningPrDiff bar  press_max_gauge=0.2 MPa  area_max=HydFcnParams.checkValves.maxOpeningArea mm^2  area_leak="HydFcnParams.checkValves.leakageArea  mm^2"  p_diff_TLU=[0.01 : 0.01 : 0.1] MPa  valve_area_TLU=[1e-10, 1e-05, 2e-05, 3e-05, 4e-05, 5e-05, 6e-05, 7.5e-05, 8.5e-05, .0001] m^2  vol_flow_TLU=[.000358, .045, .11, .191, .284, .39, .505, .63, .764, .905] .* 1e-3 m^3/s  area=inf m^2  Cd=HydFcnParams.checkValves.dischargeCoef  Re_c=HydFcnParams.checkValves.critReynoldsNmbr  smoothing_factor=HydFcnParams.checkValves.smoothingFactor  pressure_recovery=simscape.enum.onoff.off  opening_dynamics=simscape.enum.onoff.off  tau=0.1 s
  CVC GerotorA : fl_lib/Isothermal Liquid/Elements/Constant Volume Chamber (IL)  volume=HydFcnParams.steerValve.gerChamberVol mm^3  p_I_specify=off  p_I_priority=High  p_I=0.101325 MPa  p_I_nominal_specify=off  p_I_nominal_value=1  p_I_nominal_unit=MPa
  CVC GerotorB : fl_lib/Isothermal Liquid/Elements/Constant Volume Chamber (IL)  volume=HydFcnParams.steerValve.gerChamberVol mm^3  p_I_specify=off  p_I_priority=High  p_I=0.101325 MPa  p_I_nominal_specify=off  p_I_nominal_value=1  p_I_nominal_unit=MPa
  CVC Steer A : fl_lib/Isothermal Liquid/Elements/Constant Volume Chamber (IL)  volume=HydFcnParams.steerValve.gerChamberVol mm^3  p_I_specify=off  p_I_priority=High  p_I=0.101325 MPa  p_I_nominal_specify=off  p_I_nominal_value=1  p_I_nominal_unit=MPa
  CVC Steer B : fl_lib/Isothermal Liquid/Elements/Constant Volume Chamber (IL)  volume=HydFcnParams.steerValve.gerChamberVol mm^3  p_I_specify=off  p_I_priority=High  p_I=0.101325 MPa  p_I_nominal_specify=off  p_I_nominal_value=1  p_I_nominal_unit=MPa
  Gerotor : SimscapeFluids_lib/Isothermal Liquid/Pumps & Motors/Fixed-Displacement Motor (IL)  leakage_friction_spec=fluids.isothermal_liquid.pumps_motors.enum.MotorLossSpec.InputEfficiency  displacement=HydFcnParams.steerValve.gerDisplacement cm^3/rev  omega_nominal=20 rpm  p_nominal=10 MPa  vol_eff_nominal=0.92  mech_eff_nominal=0.88  no_load_torque=0 N*m  p_diff_eff_TLU=[.1, 1, 2] MPa  omega_eff_TLU=[250, 500, 1000, 2000, 3000, 4000] rpm  vol_eff_TLU=[.816, .908, .954, .977, .981, .984; .325, .663, .831, .916, .925, .946; .137, .568, .78, .892, .893, .91]  mech_eff_TLU=[.996, .996, .996, .996, .996, .996; .988, .989, .989, .989, .989, .99; .981, .981, .982, .982, .983, .984]  p_diff_loss_TLU=[.1, 1, 2] MPa  omega_loss_TLU=[250, 500, 1000, 2000, 3000, 4000] rpm  vol_loss_TLU=1e-3 * [.023, .023, .023, .023, .0285, .032; .0844, .0842, .0845, .084, .1125, .108; .1079, .108, .11, .108, .1605, .18] m^3/s  mech_loss_TLU=[.002, .002, .002, .002, .002, .002; .0607, .0556, .0556, .0556, .0556, .0505; .1937, .1937, .1833, .1833, .1729, .1626] N*m  q_shaft_TLU=[.125, .25, .5, 1, 1.5, 2] * 1e-3 m^3/s  p_diff_shaft_TLU=[.1, 1, 2] MPa  torque_shaft_TLU=[.47, 4.72, 9.35; .47, 4.7, 9.36; .47, 4.7, 9.4; .47, 4.7, 9.41; .47, 4.7, 9.46; .47, 4.68, 9.5] N*m  omega_shaft_TLU=[205, 80, 35; 455, 330, 285; 955, 831, 780; 1950, 1830, 1780; 2940, 2775, 2680; 3940, 3780, 3640] rpm  vol_eff_min=1e-3  vol_eff_max=1  mech_eff_min=1e-3  mech_eff_max=1  pressure_threshold=1e-3 MPa  omega_threshold=100 rpm  supplied_range_check=simscape.enum.assert.action.none  motor_mode_check=simscape.enum.assert.action.none  pressure_check=simscape.enum.assert.action.none  p_min_valid=0.101325 MPa
  MRRef Gerotor : fl_lib/Mechanical/Rotational Elements/Mechanical Rotational Reference
  Orifices : Subsystem
      mask Display: image('sm_wheel_loader_valve_steer_IMAGE.png');
  PRV Steer Pump : SimscapeFluids_lib/Isothermal Liquid/Valves & Orifices/Pressure Control Valves/Pressure Relief Valve (IL)  set_pressure_spec=foundation.enum.constant_controlled.constant  opening_spec=fluids.isothermal_liquid.valves_orifices.enum.opening_spec.linear  pressure_spec=fluids.isothermal_liquid.valves_orifices.enum.pressure_control_spec.dp  p_set_gauge=0.1 MPa  p_set_differential=HydFcnParams.pumpPRV.reliefPr bar  p_range=HydFcnParams.pumpPRV.regRange bar  area_max=HydFcnParams.pumpPRV.maxOpeningArea mm^2  area_leak=HydFcnParams.pumpPRV.leakageArea mm^2  p_diff_TLU=[30.15e5 : 15e3 : 31.35e5] Pa  p_gauge_TLU=[30.15e5 : 15e3 : 31.35e5] Pa  valve_area_TLU=[1 : 1 : 9] .* 1e-5 m^2  vol_flow_TLU=[1e-09, 3.6e-05, 8.9e-05, .00015, .00023, .00031] m^3/s  area=inf m^2  Cd=HydFcnParams.pumpPRV.dischargeCoef  Re_c=HydFcnParams.pumpPRV.critReynoldsNmbr  smoothing_factor=HydFcnParams.pumpPRV.smoothingFactor  pressure_recovery=simscape.enum.onoff.off  opening_dynamics=simscape.enum.onoff.off  tau=0.1 s
  PRV SteerA : SimscapeFluids_lib/Isothermal Liquid/Valves & Orifices/Pressure Control Valves/Pressure Relief Valve (IL)  set_pressure_spec=foundation.enum.constant_controlled.constant  opening_spec=fluids.isothermal_liquid.valves_orifices.enum.opening_spec.linear  pressure_spec=fluids.isothermal_liquid.valves_orifices.enum.pressure_control_spec.dp  p_set_gauge=0.1 MPa  p_set_differential=HydFcnParams.actPRV.reliefPr bar  p_range=HydFcnParams.actPRV.regRange bar  area_max=HydFcnParams.actPRV.maxOpeningArea mm^2  area_leak=HydFcnParams.actPRV.leakageArea mm^2  p_diff_TLU=[30.15e5 : 15e3 : 31.35e5] Pa  p_gauge_TLU=[30.15e5 : 15e3 : 31.35e5] Pa  valve_area_TLU=[1 : 1 : 9] .* 1e-5 m^2  vol_flow_TLU=[1e-09, 3.6e-05, 8.9e-05, .00015, .00023, .00031] m^3/s  area=inf m^2  Cd=HydFcnParams.actPRV.dischargeCoef  Re_c=HydFcnParams.actPRV.critReynoldsNmbr  smoothing_factor=HydFcnParams.actPRV.smoothingFactor  pressure_recovery=simscape.enum.onoff.off  opening_dynamics=simscape.enum.onoff.off  tau=0.1 s
  PRV SteerB : SimscapeFluids_lib/Isothermal Liquid/Valves & Orifices/Pressure Control Valves/Pressure Relief Valve (IL)  set_pressure_spec=foundation.enum.constant_controlled.constant  opening_spec=fluids.isothermal_liquid.valves_orifices.enum.opening_spec.linear  pressure_spec=fluids.isothermal_liquid.valves_orifices.enum.pressure_control_spec.dp  p_set_gauge=0.1 MPa  p_set_differential=HydFcnParams.actPRV.reliefPr bar  p_range=HydFcnParams.actPRV.regRange bar  area_max=HydFcnParams.actPRV.maxOpeningArea mm^2  area_leak=HydFcnParams.actPRV.leakageArea mm^2  p_diff_TLU=[30.15e5 : 15e3 : 31.35e5] Pa  p_gauge_TLU=[30.15e5 : 15e3 : 31.35e5] Pa  valve_area_TLU=[1 : 1 : 9] .* 1e-5 m^2  vol_flow_TLU=[1e-09, 3.6e-05, 8.9e-05, .00015, .00023, .00031] m^3/s  area=inf m^2  Cd=HydFcnParams.actPRV.dischargeCoef  Re_c=HydFcnParams.actPRV.critReynoldsNmbr  smoothing_factor=HydFcnParams.actPRV.smoothingFactor  pressure_recovery=simscape.enum.onoff.off  opening_dynamics=simscape.enum.onoff.off  tau=0.1 s
  PS Constant : fl_lib/Physical Signals/Sources/PS Constant  constant=1
  Sleeve Damper : fl_lib/Mechanical/Rotational Elements/Rotational Damper  D=HydFcnParams.steerValve.sleeveDamping N*m*s/rad  w_specify=off  w_priority=None  w=0 rad/s  w_nominal_specify=off  w_nominal_value=1  w_nominal_unit=rad/s  t_specify=off  t_priority=None  t=0 N*m  t_nominal_specify=off  t_nominal_value=1  t_nominal_unit=N*m
  Sleeve Deflection : fl_lib/Mechanical/Mechanical Sensors/Ideal Rotational Motion Sensor  reference=foundation.enum.MeasurementReference.difference  acceleration_port=false  velocity_port=false  position_port=true  wrap_angle=false  offset=0 rad
  Sleeve Hard Stop : fl_lib/Mechanical/Rotational Elements/Rotational Hard Stop  upper_bnd=HydFcnParams.steerValve.maxRelAngle rad  lower_bnd=HydFcnParams.steerValve.minRelAngle rad  model=simscape.enum.hardstop.smooth  stiff_up=HydFcnParams.steerValve.hardstopStiff N*m/rad  stiff_low=HydFcnParams.steerValve.hardstopStiff N*m/rad  D_up=HydFcnParams.steerValve.hardstopDamping N*m*s/rad  D_low=HydFcnParams.steerValve.hardstopDamping N*m*s/rad  transition=0.0001 rad  coeff_rest=0.7  w_tol=0.1 rad/s  trq_tol=0.001 N*m  w_specify=off  w_priority=None  w=0 rad/s  w_nominal_specify=off  w_nominal_value=1  w_nominal_unit=rad/s  t_specify=off  t_priority=None  t=0 N*m  t_nominal_specify=off  t_nominal_value=1  t_nominal_unit=N*m  phi_specify=off  phi_priority=High  phi=0 rad  phi_nominal_specify=off  phi_nominal_value=1  phi_nominal_unit=rad  M_specify=off  M_priority=None  M=0
  Sleeve Inertia : fl_lib/Mechanical/Rotational Elements/Inertia  inertia=0.01*10 kg*m^2  num_ports=foundation.enum.numPorts2.two  w_specify=off  w_priority=High  w=0 rad/s  w_nominal_specify=off  w_nominal_value=1  w_nominal_unit=rad/s  t_specify=off  t_priority=None  t=0 N*m  t_nominal_specify=off  t_nominal_value=1  t_nominal_unit=N*m
  Sleeve Spring : fl_lib/Mechanical/Rotational Elements/Rotational Spring  spr_rate=HydFcnParams.steerValve.sleeveSpringStiff N*m/rad  w_specify=off  w_priority=None  w=0 rad/s  w_nominal_specify=off  w_nominal_value=1  w_nominal_unit=rad/s  t_specify=off  t_priority=None  t=0 N*m  t_nominal_specify=off  t_nominal_value=1  t_nominal_unit=N*m  phi_specify=off  phi_priority=High  phi=0 rad  phi_nominal_specify=off  phi_nominal_value=1  phi_nominal_unit=rad
  qSleeve to xSpool : Subsystem
  P : PMIOPort  Side=Left
  T : PMIOPort  Port=2  Side=Left
  A : PMIOPort  Port=3  Side=Right
  B : PMIOPort  Port=4  Side=Right
  SW : PMIOPort  Port=5  Side=Left
  connections:
  CV SteerB/RConn1 -- PRV SteerB/LConn1 -- Orifices/RConn4 -- B/RConn1 -- CVC Steer B/LConn1
  A/RConn1 -- CVC Steer A/LConn1 -- PRV SteerA/LConn1 -- CV SteerA/RConn1 -- Orifices/RConn1
  P/RConn1 -- CV SteerP/LConn1 -- PRV Steer Pump/LConn1
  PRV SteerA/RConn1 -- CV SteerA/LConn1 -- Orifices/LConn3 -- T/RConn1 -- PRV Steer Pump/RConn1 -- PRV SteerB/RConn1 -- CV SteerB/LConn1
  CV SteerP/RConn1 -- Orifices/LConn2
  Orifices/LConn1 -- qSleeve to xSpool/RConn1
  PS Constant/RConn1 -- Gerotor/LConn2 -- Gerotor/LConn1
  Gerotor/RConn3 -- Orifices/RConn3 -- CVC GerotorB/LConn1
  MRRef Gerotor/LConn1 -- Gerotor/RConn2
  Sleeve Inertia/RConn1 -- Gerotor/RConn1
  Gerotor/LConn3 -- CVC GerotorA/LConn1 -- Orifices/RConn2
  Sleeve Spring/RConn1 -- Sleeve Deflection/RConn1 -- Sleeve Hard Stop/RConn1 -- Sleeve Damper/RConn1 -- SW/RConn1
  Sleeve Hard Stop/LConn1 -- Sleeve Deflection/LConn1 -- Sleeve Inertia/LConn1 -- Sleeve Spring/LConn1 -- Sleeve Damper/LConn1
  qSleeve to xSpool/LConn1 -- Sleeve Deflection/RConn2
